simulink model "LIB_CoffeeMachine"  (R2019a)
settings: Solver=FixedStepAuto  StartTime=0.0  StopTime=10.0  FixedStep=0.025  RelTol=1e-3
libraries: simulink_extras x1
settings Model: SimulationMode=external  Creator=RAPQ2Y  LastModifiedBy=RAPQ2Y
settings HardwareCC: ProdBitPerPointer=32  ProdBitPerSizeT=32  ProdBitPerPtrDiffT=32  ProdWordSize=32  ProdLongLongMode=on  ProdHWDeviceType=PHOENIX CONTACT->Generic PLCnext 32bit  TargetPreprocMaxBitsSint=64  TargetPreprocMaxBitsUint=64
settings SFSimCC: MATLABDynamicMemAlloc=off
settings RTWCC: SystemTargetFile=pxc_plcn.tlc  TLCOptions=-p10000000000000000000  TemplateMakefile=pxc_plcn__2019a.tmf  Description=PLCnext Target for Simulink  TargetLang=C++
settings CodeAppCC: MaxIdLength=63
settings STFCustomTargetCC: TargetLibSuffix=.a  TargetLangStandard=C++03 (ISO)  ParMdlRefBuildCompliant=on  ConcurrentExecutionCompliant=on  CombineOutputUpdateFcns=on  GRTInterface=off  SystemTargetFile=pxc_plcn.tlc
settings GRTTargetCC: TargetLibSuffix=.a  TargetLangStandard=C++03 (ISO)  CompOptLevelCompliant=off  MatFileLogging=off  CPPClassGenCompliant=off  UseToolchainInfoCompliant=off  ExtModeMexFile=ext_comm_plcn

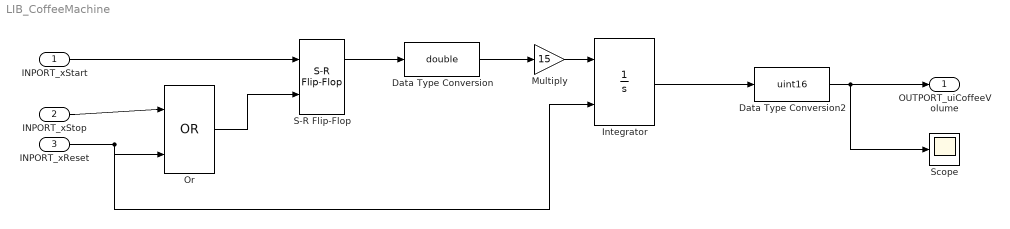
== system LIB_CoffeeMachine ==
  INPORT_xStart : Inport  OutDataTypeStr=boolean
  INPORT_xStop : Inport  Port=2  OutDataTypeStr=boolean
  INPORT_xReset : Inport  Port=3  OutDataTypeStr=boolean
  Data Type Conversion : DataTypeConversion  OutDataTypeStr=double
  Data Type Conversion2 : DataTypeConversion  OutDataTypeStr=uint16
  Integrator : Integrator  ExternalReset=rising
  Multiply : Gain  Gain=15
  Or : Logic  Operator=OR  IconShape=distinctive  AllPortsSameDT=off  OutDataTypeStr=boolean
  S-R Flip-Flop : simulink_extras/Flip Flops/S-R Flip-Flop  initial_condition=0
  Scope : Scope
  OUTPORT_uiCoffeeVolume : Outport  OutDataTypeStr=uint16
  wires:
  INPORT_xStop/1 -> Or/1
  INPORT_xStart/1 -> S-R Flip-Flop/1
  INPORT_xReset/1 -> Integrator/2, Or/2
  Or/1 -> S-R Flip-Flop/2
  S-R Flip-Flop/1 -> Data Type Conversion/1
  Data Type Conversion/1 -> Multiply/1
  Data Type Conversion2/1 -> Scope/1, OUTPORT_uiCoffeeVolume/1
  Integrator/1 -> Data Type Conversion2/1
  Multiply/1 -> Integrator/1
